simulink model "ME4564_Hw4"  (R2021a)
settings: Solver=VariableStepAuto  StartTime=0.0  StopTime=T  RelTol=1e-3
model workspace (MAT data in the model file):
  T = 80
  V0_lead = 25
  V0_trail = 20
  X0_lead = 50
  X0_trail = 10
undefined symbols (not defined in the file): Ts
libraries: slpidlib x1
settings Model: Creator=Sam Kramer  LastModifiedBy=Sam Kramer

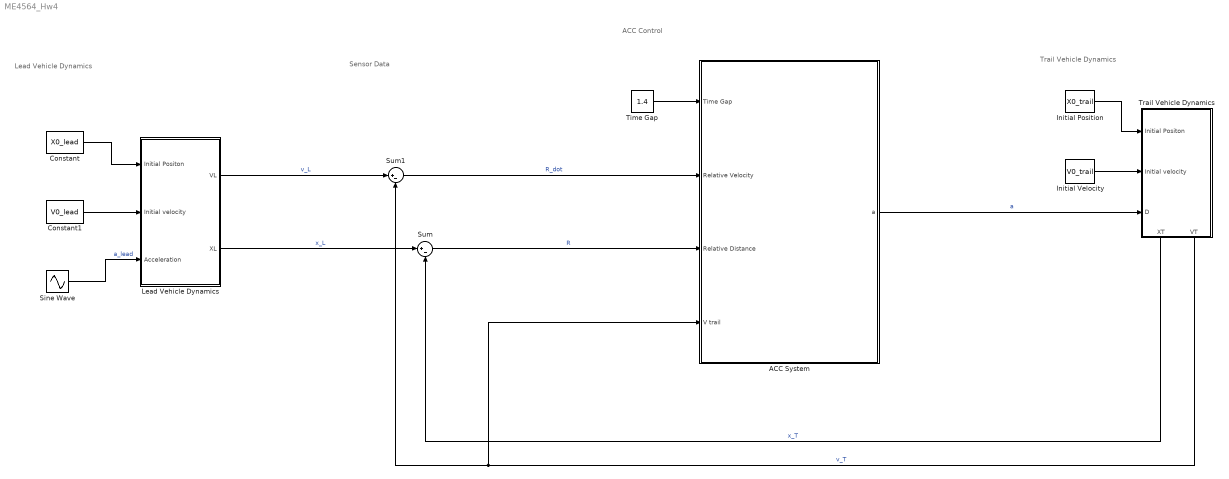
== system ME4564_Hw4 ==
  note: Trail Vehicle Dynamics
  note: ACC Control
  note: Sensor Data
  note: Lead Vehicle Dynamics
  ACC System : Subsystem
  Constant : Constant  Value=X0_lead
  Constant1 : Constant  Value=V0_lead
  Initial Position : Constant  Value=X0_trail
  Initial Velocity : Constant  Value=V0_trail
  "Lead Vehicle Dynamics " : Subsystem
  Sine Wave : Sin  Amplitude=0.6  Frequency=0.2  SampleTime=Ts
  Sum : Sum  Inputs=|+-
  Sum1 : Sum  Inputs=|+-
  Time Gap : Constant  Value=1.4
  Trail Vehicle Dynamics : Subsystem
      settings: PortSchema="{\"entries\":[{\"content\":{\"sides\":[{\"content\":{\"connectorIds\":[\"In1\",\"In2\",\"In3\"]},\"type\":\"ConnectorPlacement.EquallySpacedRectSide\",\"uuid\":\"ff3b3543-e2c3-4a4f-aed5-bc03d577e165\"},{\"content\":{\"connectorIds\":[],\"side\":\"RIGHT\"},\"type\":\"ConnectorPlacement.EquallySpacedRectSide\",\"uuid\":\"dfc4c8fe-b627-4d3f-86c8-6fbf3cdc54bf\"},{\"content\":{\"connectorIds\":[],\"side\":\"TOP\"},\"type\":\"ConnectorPlacement.EquallySpacedRectSide\",\"uuid\":\"e3799288-102d-4a3c-a7ba-d6840a9ace01\"},{\"content\":{\"connectorIds\":[\"Out1\",\"Out2\"],\"side\":\"BOTTOM\"},\"type\":\"ConnectorPlacement.EquallySpacedRectSide\",\"uuid\":\"dc286326-63a8-45a2-bec2-a00a9bc9ce59\"}]},\"type\":\"ConnectorPlacement.EquallySpacedConnector\",\"uuid\":\"4824d044-83aa-4eca-ae9e-b586e9cb07ec\"}],\"packageUris\":[\"http://schema.mathworks.com/mf0/Connector/R2020b\"],\"version\":\"1.0\"}"
  wires:
  Time Gap/1 -> ACC System/1(Time Gap)
  Sum/1 -> ACC System/3(Relative Distance)  "R"
  Sum1/1 -> ACC System/2(Relative Velocity)  "R_dot"
  Trail Vehicle Dynamics/2(VT) -> ACC System/4(V trail), Sum1/2  "v_T"
  Trail Vehicle Dynamics/1(XT) -> Sum/2  "x_T"
  ACC System/1(a) -> Trail Vehicle Dynamics/3(D)  "a"
  "Lead Vehicle Dynamics "/1(VL) -> Sum1/1  "v_L"
  "Lead Vehicle Dynamics "/2(XL) -> Sum/1  "x_L"
  Sine Wave/1 -> "Lead Vehicle Dynamics "/3(Acceleration)  "a_lead"
  Initial Position/1 -> Trail Vehicle Dynamics/1(Initial Positon)
  Initial Velocity/1 -> Trail Vehicle Dynamics/2(Initial velocity)
  Constant/1 -> "Lead Vehicle Dynamics "/1(Initial Positon)
  Constant1/1 -> "Lead Vehicle Dynamics "/2(Initial velocity)

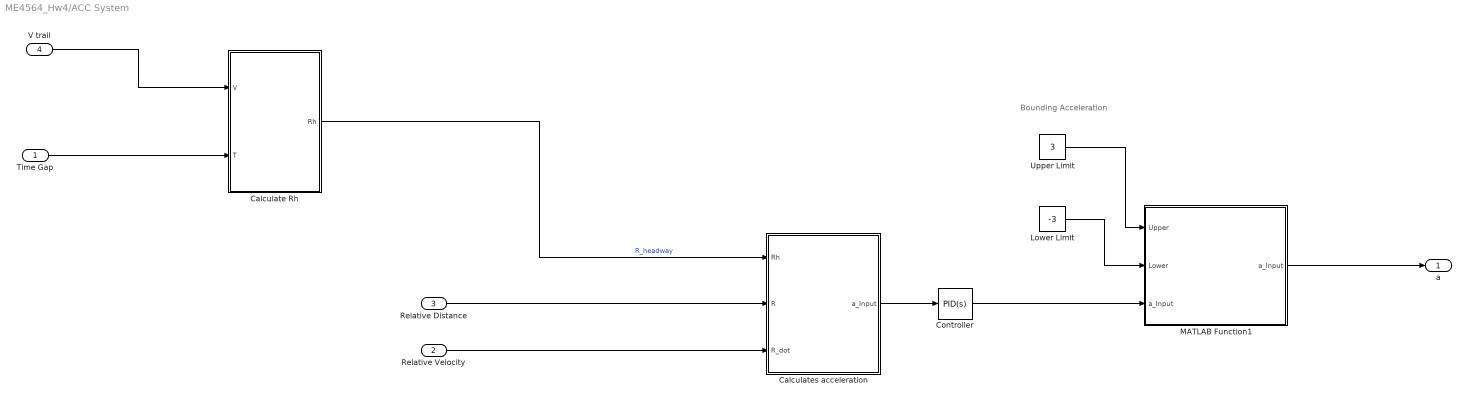
== system ME4564_Hw4/ACC System ==
  note: Bounding Acceleration
  Time Gap : Inport
  Relative Velocity : Inport  Port=2
  Relative Distance : Inport  Port=3
  V trail : Inport  Port=4
  Calculate Rh : MATLAB Function  TreatAsAtomicUnit=on
  Calculates acceleration : MATLAB Function  TreatAsAtomicUnit=on
  Controller : slpidlib/PID Controller  Controller=PID  Form=Parallel  TimeDomain=Continuous-time  UseExternalTs=off  SampleTime=-1  IntegratorMethod=Forward Euler  FilterMethod=Forward Euler  ControllerParametersSource=internal  P=1  I=-1  D=1.5  UseFilter=on  N=100  TunerSelectOption=Transfer Function Based (PID Tuner App)  InitialConditionSource=internal  InitialConditionForIntegrator=0  InitialConditionForFilter=0  DifferentiatorICPrevScaledInput=0  ExternalReset=none  TrackingMode=off  Kt=1  LimitOutput=off  SatLimitsSource=internal  UpperSaturationLimit=inf  LowerSaturationLimit=-inf  LinearizeAsGain=on  AntiWindupMode=none  Kb=1  POutMin=[]  POutMax=[]  IOutMin=[]  IOutMax=[]  DOutMin=[]  DOutMax=[]  NOutMin=[]  NOutMax=[]  SumOutMin=[]  SumOutMax=[]  SaturationOutMin=[]  SaturationOutMax=[]  PParamMin=[]  PParamMax=[]  IParamMin=[]  IParamMax=[]  DParamMin=[]  DParamMax=[]  NParamMin=[]  NParamMax=[]  KbParamMin=[]  KbParamMax=[]  KtParamMin=[]  KtParamMax=[]  KbOutMin=[]  KbOutMax=[]  KtOutMin=[]  KtOutMax=[]  IntegratorOutMin=[]  IntegratorOutMax=[]  FilterOutMin=[]  FilterOutMax=[]  SumI1OutMin=[]  SumI1OutMax=[]  SumI2OutMin=[]  SumI2OutMax=[]  SumI3OutMin=[]  SumI3OutMax=[]  SumI4OutMin=[]  SumI4OutMax=[]  SumDOutMin=[]  SumDOutMax=[]  DifferentiatorOutMin=[]  DifferentiatorOutMax=[]  FilterDiffOutCoefMin=[]  FilterDiffOutCoefMax=[]  ReciprocalOutMin=[]  ReciprocalOutMax=[]  SumDenOutMin=[]  SumDenOutMax=[]  SumNumOutMin=[]  SumNumOutMax=[]  DivideOutMin=[]  DivideOutMax=[]  UdiffTsProdOutMin=[]  UdiffTsProdOutMax=[]  NTsProdOutMin=[]  NTsProdOutMax=[]  UintegralTsProdOutMin=[]  UintegralTsProdOutMax=[]  UngainTsProdOutMin=[]  UngainTsProdOutMax=[]  IntegratorContinuousStateAttributes=''  IntegratorStateMustResolveToSignalObject=off  IntegratorRTWStateStorageClass=Auto  FilterContinuousStateAttributes=''  FilterStateMustResolveToSignalObject=off  FilterRTWStateStorageClass=Auto  ParallelPVariant=InternalParameters  IdealPVariant=Disabled  IVariant=InternalParameters  DVariant=InternalParameters  IntegratorVariant=Continuous  SatVariant=Disabled  AWVariant=Passthrough  PCopyVariant=Disabled  TRVariant=Disabled  FdbkBlocksVariant=Forward  IdealPFdbkVariant=Disabled  SatFdbkVariant=Disabled  DerivativeFilterVariant=ContFilter  NVariant=InternalParameters  NCopyVariant=Disabled  FilterICVariant=InternalICsFilter  IntegratorICVariant=InternalICs  ExternalResetVariant=Disabled  TRSumVariant=Passthrough  SumFdbkVariant=Disabled  SumVariant=Sum_PID  TsampFilterVariant=InternalTs  TsampNgainVariant=Passthrough  TsampIntegralVariant=Passthrough  ExternalSaturationOutDataTypeStr=Inherit: Same as second input
  Lower Limit : Constant  Value=-3
  MATLAB Function1 : MATLAB Function  TreatAsAtomicUnit=on
  Upper Limit : Constant  Value=3
  a : Outport
  wires:
  Calculate Rh/1(Rh) -> Calculates acceleration/1(Rh)  "R_headway"
  Time Gap/1 -> Calculate Rh/2(T)
  Relative Velocity/1 -> Calculates acceleration/3(R_dot)
  Relative Distance/1 -> Calculates acceleration/2(R)
  V trail/1 -> Calculate Rh/1(V)
  Controller/1 -> MATLAB Function1/3("a_Input ")
  MATLAB Function1/1(a_Input) -> a/1
  Upper Limit/1 -> MATLAB Function1/1(Upper)
  Lower Limit/1 -> MATLAB Function1/2(Lower)
  Calculates acceleration/1(a_Input) -> Controller/1

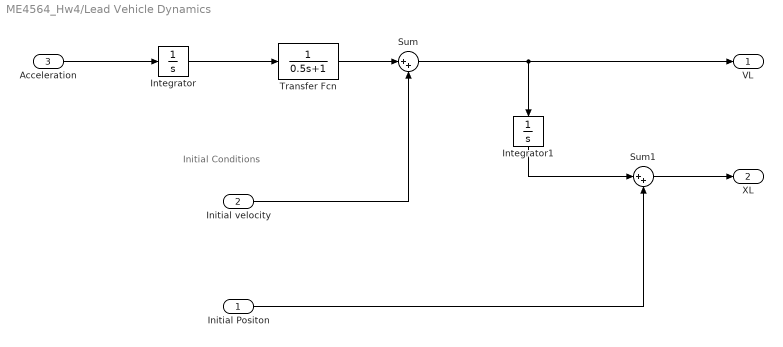
== system ME4564_Hw4/Lead Vehicle Dynamics  ==
  note: Initial Conditions
  Initial Positon : Inport
  Initial velocity : Inport  Port=2
  Acceleration : Inport  Port=3
  Integrator : Integrator
  Integrator1 : Integrator
  Sum : Sum  Inputs=|++
  Sum1 : Sum  Inputs=|++
  Transfer Fcn : TransferFcn  Denominator=[0.5 1]
  VL : Outport
  XL : Outport  Port=2
  wires:
  Integrator/1 -> Transfer Fcn/1
  Initial Positon/1 -> Sum1/2
  Sum/1 -> VL/1, Integrator1/1
  Acceleration/1 -> Integrator/1
  Integrator1/1 -> Sum1/1
  Initial velocity/1 -> Sum/2
  Transfer Fcn/1 -> Sum/1
  Sum1/1 -> XL/1

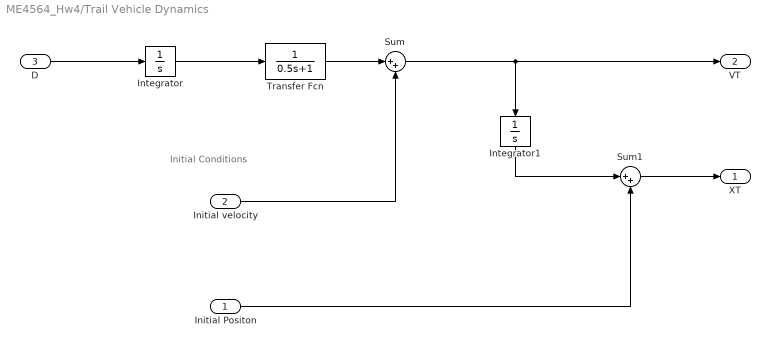
== system ME4564_Hw4/Trail Vehicle Dynamics ==
  note: Initial Conditions
  Initial Positon : Inport
  Initial velocity : Inport  Port=2
  D : Inport  Port=3
  Integrator : Integrator
  Integrator1 : Integrator
  Sum : Sum  Inputs=|++
  Sum1 : Sum  Inputs=|++
  Transfer Fcn : TransferFcn  Denominator=[0.5 1]
  XT : Outport
  VT : Outport  Port=2
  wires:
  D/1 -> Integrator/1
  Initial velocity/1 -> Sum/2
  Sum/1 -> VT/1, Integrator1/1
  Integrator1/1 -> Sum1/1
  Initial Positon/1 -> Sum1/2
  Sum1/1 -> XT/1
  Integrator/1 -> Transfer Fcn/1
  Transfer Fcn/1 -> Sum/1

== matlab function ME4564_Hw4/ACC System/Calculate Rh ==
  data: V input; T input; Rh output
function Rh = safeHeadway(V,T)
%{
    This will be the function that will calculate the safe headway based on
    speed for the vehicle using the function:
                        Rh = Rd + T*V
                Rh = Command Headway (m)
                Rd = default standstill distance (m)
                T = time gap (s)
                V = vehicle velocity
    Sam Kramer                                                      05DEC22
%}

% -- Parameters
    Rd = 1.5;     % Standstill distance (m)
    
% --Calculate Rh
    Rh = Rd + T*V;
    
end

== matlab function ME4564_Hw4/ACC System/Calculates acceleration ==
  data: Rh input; a_Input output; R input; R_dot input
function a_Input = acceleration(Rh,R,R_dot)
%{
    This will be the function that calculates the decceleration of the
    vehicle given the plase on the r'-r state space plot. A negative
    deccelleration will cause the vehicle to accelerate and vice versa.
    Uses the equation:
                        D = (R_dot^2)/(2*(R-Rh))
                R_dot = change in range (m/s)
                R = Range (m)
                Rh = Headway range (m)
    Sam Kramer                                                      06DEC22
%}
    
% --If statement
        a_Input = -(R_dot^2)/(2*(R-Rh));
end

== matlab function ME4564_Hw4/ACC System/MATLAB Function1 ==
  data: Upper input; a_Input output; Lower input; a_Input input
function a_Input = LIMITS(Upper,Lower,a_Input)
%{
    This will be the limitations for the upper and lower accelerations for
    the vehicle to prevent accelerating too fast.
    Sam Kramer                                                      06DEC22
%}

% --Acceleration Bounds

    if a_Input > Upper
        a_Input = Upper;        % Set to upper acceleration boundary
        
    elseif a_Input < Lower
        a_Input = Lower;        % Set to lower acc bound
    
    else
        % Do nothing

    end
end
